simulink model "STEVE_Simulation"  (R2024b)
settings: Solver=ode8  StartTime=0.0  StopTime=Sim.Time  FixedStep=Sim.Timestep  RelTol=1e-3  EnableMultiTasking=on
values from neighbouring files (symbols this model uses):
  AeroData = CombinedAeroData    [initialize_sim_parameters.m]
  m = 1277.9    [LQR_Controller_Design.m]    (also in controlability_analysis.m = params.mass(i); lqr_gain_scedule.m = interp_data.mass(i); matlab.mat = 974)
  q = 0.5 * rho * V^2    (= 29036.16)    [LQR_Controller_Design.m]    (also in matlab.mat = 2919.616)
  Ref_Area = RocketAeroPhysical.Reference_Area    [initialize_sim_parameters.m]
undefined symbols (not defined in the file or in its folder): Actuators, Earth, F, Initial, Light, MIL, PrelookupData, rocket_length, RocketAeroPhysical, s, ThrustLookupData, timeStep, WGS84
libraries: simulink x6, simulink_extras x4, aerolibwind2 x4, aerolibtransform2 x3, aerolibasang x3, aerolibconvert2 x2, aerolibnav x2, aerolibactuator x2, aerolibatmos2 x1, dspsrcs4 x1, mspfiltlib x1, sharedtransform x1
(part 1 of 2)
settings Model: SimulationMode=accelerator  ExtModeTrigDuration=2  Creator=jonno  LastModifiedBy=jonno
settings SolverCC: AutoInsertRateTranBlk=on
settings HardwareCC: ProdBitPerLong=64  ProdHWDeviceType=Apple->ARM64
settings RTWCC: BuildConfiguration=Faster Runs
settings GRTTargetCC: RTWCAPISignals=on  RTWCAPIParams=on

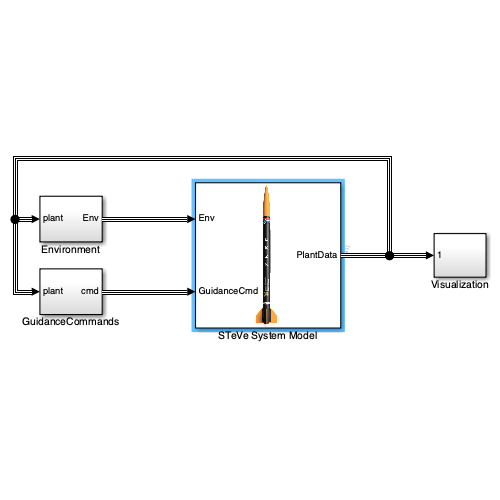
[thumbnail: Simulink's stored preview of the top-level diagram]
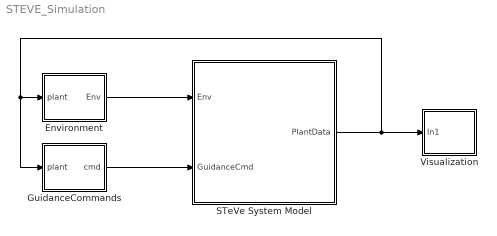
== system STEVE_Simulation ==
  Environment : Subsystem
  GuidanceCommands : Subsystem
  STeVe System Model : Subsystem
      mask Display: image('/Users/jonno/MATLAB-Drive/Rocket-Model-Simulation/STEVE_Simulator/docs/images/steve.png', [65 - (50 * (187 / 1041)), 0, 140 * (187 / 1041), 140])
  Visualization : Subsystem
  wires:
  GuidanceCommands/1(cmd) -> STeVe System Model/2(GuidanceCmd)
  Environment/1(Env) -> STeVe System Model/1(Env)
  STeVe System Model/1(PlantData) -> GuidanceCommands/1(plant), Environment/1(plant), Visualization/1(In1)

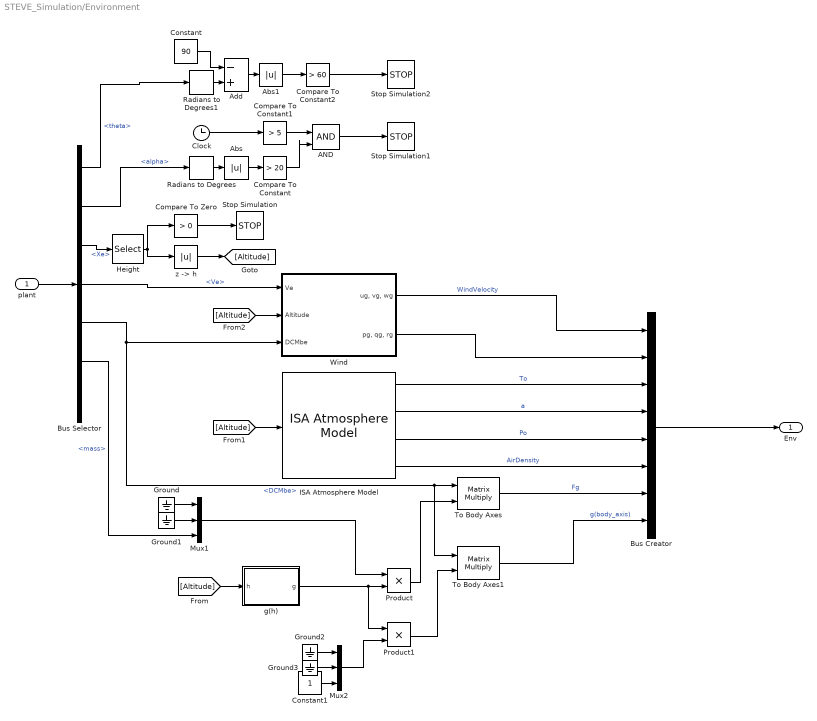
== system STEVE_Simulation/Environment ==
  plant : Inport
  AND : Logic  IconShape=distinctive  AllPortsSameDT=off  OutDataTypeStr=boolean
  Abs : Abs  SaturateOnIntegerOverflow=off
  Abs1 : Abs  SaturateOnIntegerOverflow=off
  Add : Sum  Inputs=-+
  Bus Creator : BusCreator  Inputs=8
  Bus Selector : BusSelector  OutputSignals=body angles.theta,alpha,Xe,Ve,DCMbe,mass,lat
  Clock : Clock
  Compare To Constant : simulink/Logic and Bit Operations/Compare To Constant  relop=>  const=20  OutDataTypeStr=boolean
  Compare To Constant1 : simulink/Logic and Bit Operations/Compare To Constant  relop=>  const=5  OutDataTypeStr=boolean
  Compare To Constant2 : simulink/Logic and Bit Operations/Compare To Constant  relop=>  const=60  OutDataTypeStr=boolean
  Compare To Zero : simulink/Logic and Bit Operations/Compare To Zero  relop=>  OutDataTypeStr=boolean
  Constant : Constant  Value=90
  Constant1 : Constant
  Ground{,1..3} (4 alike) : Ground
  Height : Selector  IndexMode=Zero-based  InputPortWidth=3  IndexOptions=Index vector (dialog)  Indices=2  OutputSizes=1
  ISA Atmosphere Model : aerolibatmos2/ISA Atmosphere Model  useExtended=on  action=None  custom=off  viscosityOut=off  g=9.80665  gamma=1.4  R=287.0531  L=0.0065  h_trop=11000  h_strat=20000  rho0=1.225  P0=101325  T0=288.15  h0=0  S=110.4  Tref=273.15  muref=1.716e-5
  Mux1 : Mux  Inputs=3
  Mux2 : Mux  Inputs=3
  Product : Product
  Product1 : Product
  Radians to Degrees : simulink_extras/Transformations/Radians to Degrees
  Radians to Degrees1 : simulink_extras/Transformations/Radians to Degrees
  Stop Simulation : Stop
  Stop Simulation1 : Stop
  Stop Simulation2 : Stop
  To Body Axes : Product  Multiplication=Matrix(*)
  To Body Axes1 : Product  Multiplication=Matrix(*)
  Wind : Subsystem
  g(h) : MATLAB Function  TreatAsAtomicUnit=on
  "z -> h" : Abs  SaturateOnIntegerOverflow=off
  Env : Outport
  wires:
  plant/1 -> Bus Selector/1
  Bus Creator/1 -> Env/1
  Bus Selector/3 -> Height/1  "<Xe>"
  Height/1 -> Compare To Zero/1, "z -> h"/1
  "z -> h"/1 -> [Altitude]
  Bus Selector/6 -> Mux1/3  "<mass>"
  Ground/1 -> Mux1/1
  Ground1/1 -> Mux1/2
  Bus Selector/5 -> Wind/3(DCMbe), To Body Axes1/1, To Body Axes/1  "<DCMbe>"
  [Altitude] -> ISA Atmosphere Model/1
  To Body Axes/1 -> Bus Creator/7  "Fg"
  ISA Atmosphere Model/4 -> Bus Creator/6  "AirDensity"
  ISA Atmosphere Model/3 -> Bus Creator/5  "Po"
  ISA Atmosphere Model/2 -> Bus Creator/4  "a"
  ISA Atmosphere Model/1 -> Bus Creator/3  "To"
  Bus Selector/4 -> Wind/1(Ve)  "<Ve>"
  [Altitude] -> Wind/2(Altitude)
  Wind/2("pg, qg, rg") -> Bus Creator/2
  Mux1/1 -> Product/1
  Product/1 -> To Body Axes/2
  [Altitude] -> g(h)/1(h)
  g(h)/1(g) -> Product1/1, Product/2
  Wind/1("ug, vg, wg") -> Bus Creator/1  "WindVelocity"
  Bus Selector/2 -> Radians to Degrees/1  "<alpha>"
  Compare To Zero/1 -> Stop Simulation/1
  AND/1 -> Stop Simulation1/1
  Compare To Constant/1 -> AND/2
  Compare To Constant1/1 -> AND/1
  Clock/1 -> Compare To Constant1/1
  Radians to Degrees/1 -> Abs/1
  Abs/1 -> Compare To Constant/1
  Bus Selector/1 -> Radians to Degrees1/1  "<theta>"
  Radians to Degrees1/1 -> Add/2
  Constant/1 -> Add/1
  Add/1 -> Abs1/1
  Abs1/1 -> Compare To Constant2/1
  Compare To Constant2/1 -> Stop Simulation2/1
  Ground2/1 -> Mux2/1
  Ground3/1 -> Mux2/2
  Constant1/1 -> Mux2/3
  Mux2/1 -> Product1/2
  Product1/1 -> To Body Axes1/2
  To Body Axes1/1 -> Bus Creator/8  "g(body_axis)"

== system STEVE_Simulation/GuidanceCommands ==
  plant : Inport
  Add : Sum  Inputs=+++
  Bus Creator : BusCreator  Inputs=2
  Constant : Constant  Value=85
  Degrees to Radians : simulink_extras/Transformations/Degrees to Radians
  Rate Limiter : RateLimiter  RisingSlewLimit=Initial.Conditions.pitchRate  FallingSlewLimit=-Initial.Conditions.pitchRate  SampleTimeMode=inherited
  Rate Limiter1 : RateLimiter  RisingSlewLimit=20  FallingSlewLimit=-20  SampleTimeMode=inherited
  Rate Limiter2 : RateLimiter  RisingSlewLimit=0.1  FallingSlewLimit=-0.1  SampleTimeMode=inherited
  Rate Limiter3 : RateLimiter  SampleTimeMode=inherited
  Scope : Scope
  ThetaCmd : Step  Time=8  After=90 - Initial.Conditions.tiltAngle*180/pi  SampleTime=0
  ThetaCmd1 : Step  Time=0.5  Before=90  After=Initial.Conditions.tiltAngle*180/pi  SampleTime=0
  ThetaCmd2 : Step  Time=65  After=0  SampleTime=0
  ThrottleCmd %1 : Step  Time=Actuators.Engine.BurnTime  Before=1  After=0.05  SampleTime=0  VectorParams1D=off
  To Workspace : ToWorkspace  VariableName=thetaCmd  SaveFormat=Timeseries  SampleTime=-1
  cmd : Outport
  wires:
  Bus Creator/1 -> cmd/1
  ThetaCmd/1 -> Rate Limiter/1  "ThetaCmd"
  Degrees to Radians/1 -> Scope/1, To Workspace/1, Bus Creator/2  "ThetaCmd"
  ThrottleCmd %1/1 -> Rate Limiter2/1  "ThrottleCmd"
  Rate Limiter/1 -> Add/1
  ThetaCmd1/1 -> Rate Limiter1/1  "ThetaCmd"
  Rate Limiter1/1 -> Add/2
  Rate Limiter2/1 -> Bus Creator/1  "ThrottleCmd"
  ThetaCmd2/1 -> Rate Limiter3/1  "ThetaCmd"
  Rate Limiter3/1 -> Add/3
  Constant/1 -> Degrees to Radians/1

== system STEVE_Simulation/STeVe System Model ==
  Env : Inport
  GuidanceCmd : Inport  Port=2
  Avionics : Subsystem
  Env1 : InportShadow
  Flight Sensors : Subsystem
  Vehicle Dynamics : Subsystem
  PlantData : Outport
  wires:
  Env/1 -> Vehicle Dynamics/1(Env)
  Vehicle Dynamics/1(PlantData) -> Flight Sensors/2(Plant), Avionics/3(PlantData), PlantData/1  "Plant"
  Avionics/1(ActCmd) -> Vehicle Dynamics/2(ActCmd)
  GuidanceCmd/1 -> Avionics/1(GuidanceCommandBus)
  Env1/1 -> Flight Sensors/1(Env)
  Flight Sensors/1(Sensors) -> Avionics/2(Sensors)

== system STEVE_Simulation/Visualization ==
  In1 : Inport
  Bus Selector : BusSelector  OutputSignals=Xe
  Bus Selector1 : BusSelector  OutputSignals=Ve,Xe,Vb,body angles.phi,body angles.theta,body angles.psi,alpha,lat,long,alt,w
  Demux : Demux  Outputs=3
  In2 : InportShadow
  Multiply : Gain  Gain=-1
  To Workspace : ToWorkspace  VariableName=Ve  SaveFormat=Timeseries  SampleTime=-1
  To Workspace1 : ToWorkspace  VariableName=Xe  SaveFormat=Timeseries  SampleTime=-1
  To Workspace10 : ToWorkspace  VariableName=w  SaveFormat=Timeseries  SampleTime=-1
  To Workspace2 : ToWorkspace  VariableName=Vb  SaveFormat=Timeseries  SampleTime=-1
  To Workspace3 : ToWorkspace  VariableName=phi  SaveFormat=Timeseries  SampleTime=-1
  To Workspace4 : ToWorkspace  VariableName=theta  SaveFormat=Timeseries  SampleTime=-1
  To Workspace5 : ToWorkspace  VariableName=psi  SaveFormat=Timeseries  SampleTime=-1
  To Workspace6 : ToWorkspace  VariableName=alpha  SaveFormat=Timeseries  SampleTime=-1
  To Workspace7 : ToWorkspace  VariableName=lat  SaveFormat=Timeseries  SampleTime=-1
  To Workspace8 : ToWorkspace  VariableName=long  SaveFormat=Timeseries  SampleTime=-1
  To Workspace9 : ToWorkspace  VariableName=alt  SaveFormat=Timeseries  SampleTime=-1
  XY Graph : Record  FileSettingsInternal="{\"entries\":[{\"content\":{\"excelSettings\":{\"content\":{},\"type\":\"Streamout.ExcelSettings\"}},\"type\":\"Streamout.FileSettingStorage\",\"uuid\":\"\"}],\"packageUris\":[\"http:\\/\\/schema.mathworks.com\\/mf0\\/streamout_blocks\\/R2020a\"],\"version\":\"1.0\"}"  Layout=[1 1]  SignalsInternal="{\"entries\":[{\"content\":{\"signals\":[{\"content\":{\"blockPath\":[],\"dimensions\":[1],\"domain\":\"\",\"lineColor\":\"#a2142f\",\"plots\":[ 1 ],\"port\":1,\"signalID\":1,\"signalName\":\"Demux:1\"},\"type\":\"RecordBlkView.Signal\",\"uuid\":\"\"},{\"content\":{\"blockPath\":[],\"dimensions\":[1],\"domain\":\"\",\"lineColor\":\"#139fff\",\"plots\":[ 1 ],\"port\":2,\"signalID\":2,\"signalName\":\"Multiply\"},\"type\":\"RecordBlkView.Signal\",\"uuid\":\"\"}]},\"type\":\"RecordBlkView.InputSignals\",\"uuid\":\"\"}],\"packageUris\":[\"http:\\/\\/schema.mathworks.com\\/mf0\\/streamout_blocks\\/R2020a\"],\"version\":\"1.0\"}"  VisualizationBindings="{\"xyplotplugin\":{\"info\":[{\"series\":[{\"bindingParametersList\":[{\"parameter\":\"X-Axis\",\"signalID\":1,\"signalName\":\"Demux:1\"},{\"parameter\":\"Y-Axis\",\"signalID\":2,\"signalName\":\"Multiply\"}],\"seriesID\":0}],\"subplotID\":1}]}}"  CompatibilityTag=XY
  wires:
  In1/1 -> Bus Selector/1
  Bus Selector/1 -> Demux/1  "<Xe>"
  Multiply/1 -> XY Graph/2
  Demux/3 -> Multiply/1
  Demux/1 -> XY Graph/1
  In2/1 -> Bus Selector1/1
  Bus Selector1/1 -> To Workspace/1  "<Ve>"
  Bus Selector1/2 -> To Workspace1/1  "<Xe>"
  Bus Selector1/3 -> To Workspace2/1  "<Vb>"
  Bus Selector1/4 -> To Workspace3/1  "<phi>"
  Bus Selector1/5 -> To Workspace4/1  "<theta>"
  Bus Selector1/6 -> To Workspace5/1  "<psi>"
  Bus Selector1/7 -> To Workspace6/1  "<alpha>"
  Bus Selector1/8 -> To Workspace7/1  "<lat>"
  Bus Selector1/9 -> To Workspace8/1  "<long>"
  Bus Selector1/10 -> To Workspace9/1  "<alt>"
  Bus Selector1/11 -> To Workspace10/1  "<w>"

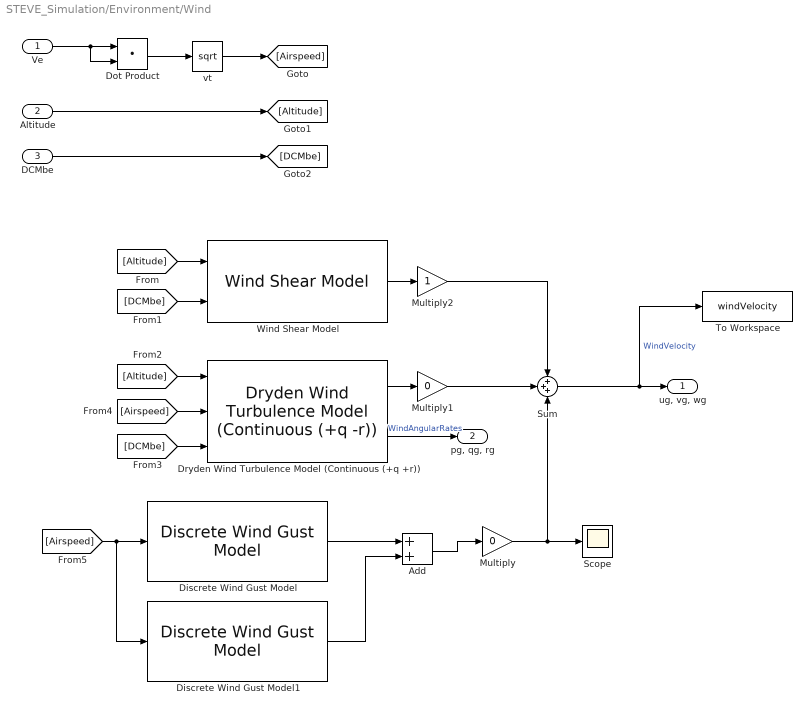
== system STEVE_Simulation/Environment/Wind ==
  Ve : Inport
  Altitude : Inport  Port=2
  DCMbe : Inport  Port=3
  Add : Sum
  Discrete Wind Gust Model : aerolibwind2/Discrete Wind Gust Model  units=Metric (MKS)  Gx=on  Gy=on  Gz=on  t_0=1  d_m=[2 2 5]  v_m=[0 0 -30]
  Discrete Wind Gust Model1 : aerolibwind2/Discrete Wind Gust Model  units=Metric (MKS)  Gx=on  Gy=on  Gz=on  t_0=2  d_m=[2 2 5]  v_m=[0 0 30]
  Dot Product : DotProduct  OutDataTypeStr=Inherit: Inherit via internal rule
  Dryden Wind Turbulence Model (Continuous (+q +r)) : aerolibwind2/Dryden Wind Turbulence Model  (Continuous (+q -r))  units=Metric (MKS)  spec=MIL-F-8785C  model=Continuous Dryden (+q +r)  W20=15  Wdeg=0  TurbProb=10^-2 - Light  L_high=533.4  Wingspan=10  ts=0.1  Seed=[23341 23342 23343 23344]  T_on=off
      settings: LibrarySourceBlock=|
      | aerolibwind2/Dryden Wind Turbulence Model
      | (Continuous (+q +r))
  Multiply : Gain  Gain=0
  Multiply1 : Gain  Gain=0
  Multiply2 : Gain
  Scope : Scope
  Sum : Sum  Inputs=+++
  To Workspace : ToWorkspace  VariableName=windVelocity  SaveFormat=Timeseries  SampleTime=-1
  Wind Shear Model : aerolibwind2/Wind Shear Model  units=Metric (MKS)  phase=Category C - Terminal Flight Phase  W_20=Wind.shear  Wdeg=90
  vt : Sqrt
  "ug, vg, wg" : Outport
  "pg, qg, rg" : Outport  Port=2
  wires:
  Ve/1 -> Dot Product/2, Dot Product/1
  Dot Product/1 -> vt/1
  vt/1 -> [Airspeed]
  DCMbe/1 -> [DCMbe]
  [Altitude] -> Wind Shear Model/1
  [DCMbe] -> Wind Shear Model/2
  [Altitude] -> Dryden Wind Turbulence Model (Continuous (+q +r))/1
  [DCMbe] -> Dryden Wind Turbulence Model (Continuous (+q +r))/3
  [Airspeed] -> Dryden Wind Turbulence Model (Continuous (+q +r))/2
  [Airspeed] -> Discrete Wind Gust Model1/1, Discrete Wind Gust Model/1
  Discrete Wind Gust Model/1 -> Add/1
  Sum/1 -> To Workspace/1, "ug, vg, wg"/1  "WindVelocity"
  Dryden Wind Turbulence Model (Continuous (+q +r))/2 -> "pg, qg, rg"/1  "WindAngularRates"
  Altitude/1 -> [Altitude]
  Multiply/1 -> Sum/3, Scope/1
  Wind Shear Model/1 -> Multiply2/1
  Dryden Wind Turbulence Model (Continuous (+q +r))/1 -> Multiply1/1
  Multiply1/1 -> Sum/2
  Multiply2/1 -> Sum/1
  Discrete Wind Gust Model1/1 -> Add/2
  Add/1 -> Multiply/1

== system STEVE_Simulation/STeVe System Model/Avionics ==
  GuidanceCommandBus : Inport
  Sensors : Inport  Port=2
  PlantData : Inport  Port=3
  Bus Selector : BusSelector  OutputSignals=Ve,body angles.theta,w
  Compare To Zero : simulink/Logic and Bit Operations/Compare To Zero  relop=>  OutDataTypeStr=boolean
  ControlSystem : Subsystem
  Delay : Delay  DelayLength=10
  Selector : Selector  InputPortWidth=3  IndexOptions=Index vector (dialog)  Indices=3  OutputSizes=1
  Stop Simulation : Stop
  ActCmd : Outport
  wires:
  PlantData/1 -> Bus Selector/1, ControlSystem/1(AvionicsBus)
  GuidanceCommandBus/1 -> ControlSystem/2(Guidance)
  ControlSystem/1(cmd) -> ActCmd/1
  Sensors/1 -> ?
  Bus Selector/1 -> Selector/1  "<Ve>"
  Selector/1 -> Compare To Zero/1
  Compare To Zero/1 -> Delay/1
  Delay/1 -> Stop Simulation/1

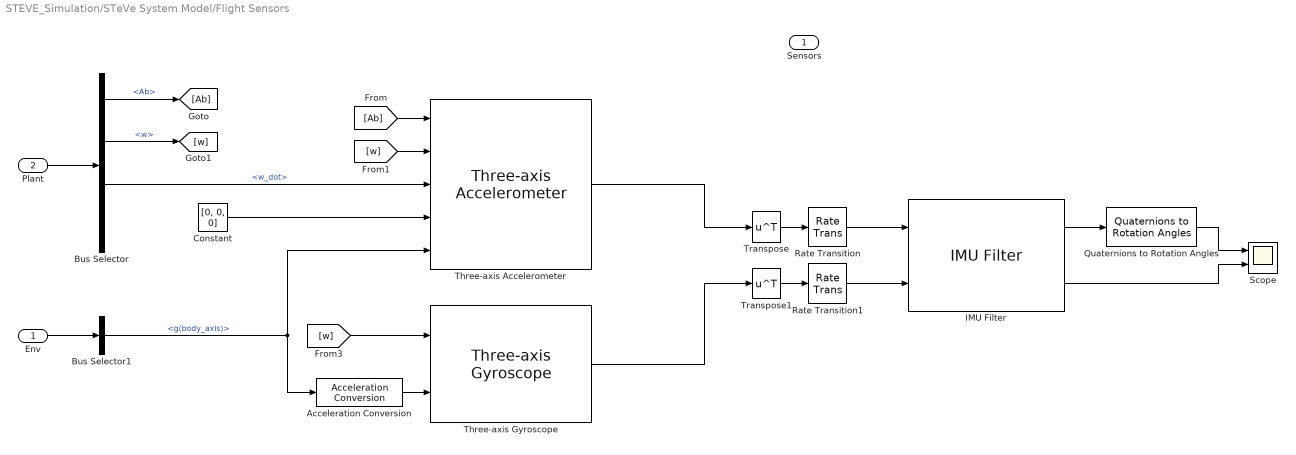
== system STEVE_Simulation/STeVe System Model/Flight Sensors ==
  Env : Inport
  Plant : Inport  Port=2
  Acceleration Conversion : aerolibconvert2/Acceleration Conversion  IU=m/s^2  OU=G's
  Bus Selector : BusSelector  OutputSignals=Ab,w,w_dot,DCMbe
  Bus Selector1 : BusSelector  OutputSignals=g(body_axis)
  Constant : Constant  Value=[0, 0, 0]
  IMU Filter : mspfiltlib/IMU Filter  DispRefFrame=NED  OrientationFormat=quaternion  DecimationFactor=1  InitialProcessNoise=imufilter.defaultProcessNoise  AccelerometerNoise=0.0001924722  GyroscopeNoise=9.1385e-5  GyroscopeDriftNoise=3.0462e-13  LinearAccelerationNoise=0.0096236100000000012  LinearAccelerationDecayFactor=0.5  SimulateUsing=Interpreted execution
  Quaternions to Rotation Angles : sharedtransform/Quaternions to Rotation Angles  rotationOrder=ZYX  aMode=aMode
  Rate Transition : RateTransition
  Rate Transition1 : RateTransition
  Scope : Scope  NumInputPorts=2
  Three-axis Accelerometer : aerolibnav/Three-axis Accelerometer  units=Metric (MKS)  acc=[0 0 0]  gtype=on  dtype_a=on  w_a=190  z_a=0.707  a_sf_cc=[1 0 0; 0 1 0; 0 0 1]  a_bias=[0 0 0]  a_Ts=0  a_rand=off  a_seeds=[23093 23094 23095]  a_pow=[0.001 0.001 0.001]  a_sat="[-inf  -inf  -inf  inf inf inf]"
  Three-axis Gyroscope : aerolibnav/Three-axis Gyroscope  dtype_g=on  w_g=190  z_g=0.707  g_sf_cc=[1 0 0; 0 1 0; 0 0 1]  g_bias=[0 0 0]  g_sen=[0 0 0]  g_Ts=0  g_rand=off  g_seeds=[23093 23094 23095]  g_pow=[0.0001 0.0001 0.0001]  g_sat="[-inf  -inf  -inf  inf inf inf]"
  Transpose : Math  Operator=transpose
  Transpose1 : Math  Operator=transpose
  Sensors : Outport
  wires:
  Plant/1 -> Bus Selector/1
  Bus Selector/1 -> [Ab]  "<Ab>"
  Bus Selector/2 -> [w]  "<w>"
  Bus Selector/3 -> Three-axis Accelerometer/3  "<w_dot>"
  Constant/1 -> Three-axis Accelerometer/4
  Env/1 -> Bus Selector1/1
  Bus Selector1/1 -> Acceleration Conversion/1, Three-axis Accelerometer/5  "<g(body_axis)>"
  [Ab] -> Three-axis Accelerometer/1
  [w] -> Three-axis Accelerometer/2
  [w] -> Three-axis Gyroscope/1
  Acceleration Conversion/1 -> Three-axis Gyroscope/2
  Three-axis Accelerometer/1 -> Transpose/1
  Three-axis Gyroscope/1 -> Transpose1/1
  Transpose/1 -> Rate Transition/1
  Transpose1/1 -> Rate Transition1/1
  Rate Transition/1 -> IMU Filter/1
  Rate Transition1/1 -> IMU Filter/2
  IMU Filter/2 -> Scope/2
  IMU Filter/1 -> Quaternions to Rotation Angles/1
  Quaternions to Rotation Angles/1 -> Scope/1

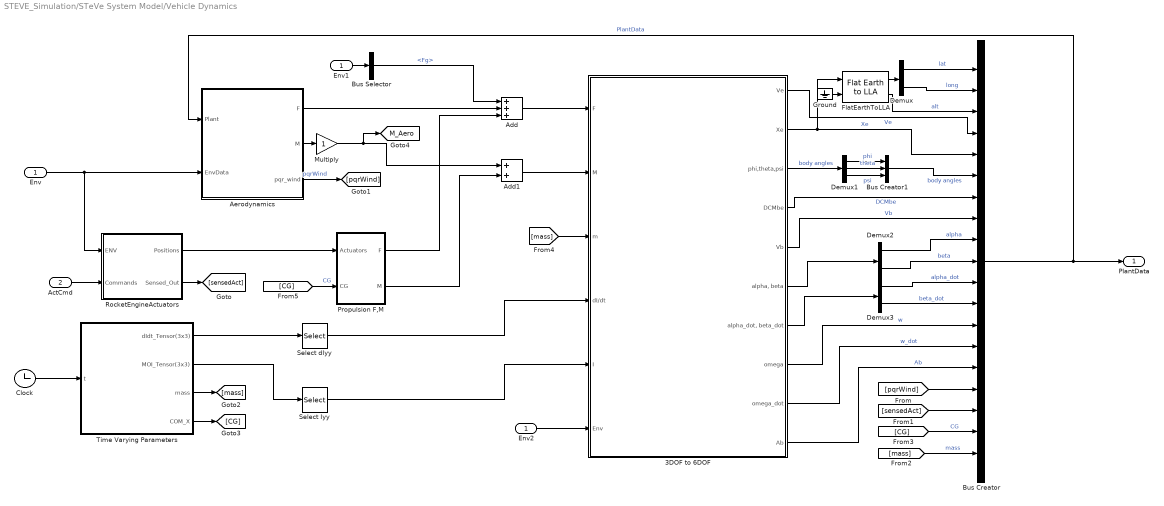
== system STEVE_Simulation/STeVe System Model/Vehicle Dynamics ==
  Env : Inport
  ActCmd : Inport  Port=2
  3DOF to 6DOF : Subsystem
  Add : Sum  Inputs=+++
  Add1 : Sum
  Aerodynamics : Subsystem
  Bus Creator : BusCreator  Inputs=19
  Bus Creator1 : BusCreator  Inputs=3
  Bus Selector : BusSelector  OutputSignals=Fg
  Clock : Clock
  Demux : Demux  Outputs=2
  Demux1 : Demux  Outputs=3
  Demux2 : Demux  Outputs=2
  Demux3 : Demux  Outputs=2
  Env1 : InportShadow
  Env2 : InportShadow
  FlatEarthToLLA : aerolibtransform2/Flat Earth to LLA  units=Metric (MKS)  ptype=Earth (WGS84)  F=1/298.257223563  R=6378137  refPosPort=off  LL0=[0 10]  psi=0
  Ground : Ground
  Multiply : Gain
  Propulsion F,M : Subsystem
  RocketEngineActuators : Subsystem
  Select Iyy : Selector  NumberOfDimensions=2  InputPortWidth=3  IndexOptions=Index vector (dialog),Index vector (dialog)  Indices=[1],[1]  OutputSizes=1,1
  Select dIyy : Selector  NumberOfDimensions=2  InputPortWidth=3  IndexOptions=Index vector (dialog),Index vector (dialog)  Indices=[1],[1]  OutputSizes=1,1
  Time Varying Parameters : Subsystem
  PlantData : Outport
  tag scope: M_Aero=global
  wires:
  ActCmd/1 -> RocketEngineActuators/2(Commands)
  RocketEngineActuators/1(Positions) -> Propulsion F,M/1(Actuators)
  Bus Creator/1 -> Aerodynamics/1(Plant), PlantData/1  "PlantData"
  3DOF to 6DOF/2(Xe) -> FlatEarthToLLA/1, Bus Creator/5  "Xe"
  Demux/1 -> Bus Creator/1  "lat"
  Demux/2 -> Bus Creator/2  "long"
  FlatEarthToLLA/1 -> Demux/1
  FlatEarthToLLA/2 -> Bus Creator/3  "alt"
  Ground/1 -> FlatEarthToLLA/2
  3DOF to 6DOF/1(Ve) -> Bus Creator/4  "Ve"
  3DOF to 6DOF/3(phi,theta,psi) -> Demux1/1  "body angles"
  Demux1/1 -> Bus Creator1/1  "phi"
  Demux1/2 -> Bus Creator1/2  "theta"
  Demux1/3 -> Bus Creator1/3  "psi"
  Bus Creator1/1 -> Bus Creator/6  "body angles"
  3DOF to 6DOF/4(DCMbe) -> Bus Creator/7  "DCMbe"
  3DOF to 6DOF/5(Vb) -> Bus Creator/8  "Vb"
  3DOF to 6DOF/6("alpha, beta") -> Demux2/1
  Demux2/1 -> Bus Creator/9  "alpha"
  Demux2/2 -> Bus Creator/10  "beta"
  Demux3/2 -> Bus Creator/12  "beta_dot"
  Demux3/1 -> Bus Creator/11  "alpha_dot"
  3DOF to 6DOF/7("alpha_dot, beta_dot") -> Demux3/1
  3DOF to 6DOF/8(omega) -> Bus Creator/13  "w"
  3DOF to 6DOF/9(omega_dot) -> Bus Creator/14  "w_dot"
  3DOF to 6DOF/10(Ab) -> Bus Creator/15  "Ab"
  [pqrWind] -> Bus Creator/16
  [sensedAct] -> Bus Creator/17
  RocketEngineActuators/2(Sensed_Out) -> [sensedAct]
  Aerodynamics/3(pqr_wind) -> [pqrWind]  "pqrWind"
  Propulsion F,M/1(F) -> Add/3
  [CG] -> Bus Creator/18  "CG"
  [mass] -> Bus Creator/19  "mass"
  Env1/1 -> Bus Selector/1
  Bus Selector/1 -> Add/1  "<Fg>"
  Env/1 -> RocketEngineActuators/1(ENV), Aerodynamics/2(EnvData)
  Propulsion F,M/2(M) -> Add1/2
  Clock/1 -> Time Varying Parameters/1(t)
  Time Varying Parameters/1(dIdt_Tensor(3x3)) -> Select dIyy/1
  Select dIyy/1 -> 3DOF to 6DOF/4(dI/dt)
  Time Varying Parameters/2(MOI_Tensor(3x3)) -> Select Iyy/1
  Select Iyy/1 -> 3DOF to 6DOF/5(I)
  Time Varying Parameters/3(mass) -> [mass]
  Time Varying Parameters/4(COM_X) -> [CG]
  [mass] -> 3DOF to 6DOF/3(m)
  Add1/1 -> 3DOF to 6DOF/2(M)
  Add/1 -> 3DOF to 6DOF/1(F)
  Aerodynamics/1(F) -> Add/2
  Env2/1 -> 3DOF to 6DOF/6(Env)
  [CG] -> Propulsion F,M/2(CG)  "CG"
  Aerodynamics/2(M) -> Multiply/1
  Multiply/1 -> Add1/1, [M_Aero]

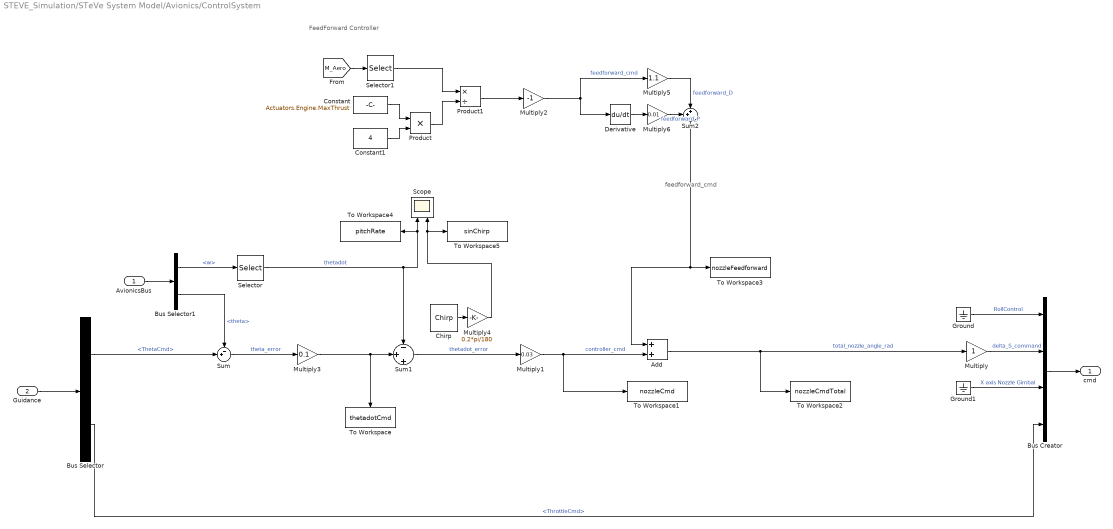
== system STEVE_Simulation/STeVe System Model/Avionics/ControlSystem ==
  note: feedforward_cmd
  note: FeedForward Controller
  AvionicsBus : Inport
  Guidance : Inport  Port=2
  Add : Sum
  Bus Creator : BusCreator  Inputs=4
  Bus Selector : BusSelector  OutputSignals=ThetaCmd,ThrottleCmd
  Bus Selector1 : BusSelector  OutputSignals=w,body angles.theta
  Chirp : dspsrcs4/Chirp  sweep=Logarithmic  mode=Unidirectional  f0=1  f1=50  t1=20  Tsweep=20  phase=0  Ts=0.0001  spf=1  datatype=double  OutputFrames=off
  Constant : Constant  Value=Actuators.Engine.MaxThrust
  Constant1 : Constant  Value=4
  Derivative : Derivative
  Ground : Ground
  Ground1 : Ground
  Multiply : Gain
  Multiply1 : Gain  Gain=0.03
  Multiply2 : Gain  Gain=-1
  Multiply3 : Gain  Gain=0.1
  Multiply4 : Gain  Gain=0.2*pi/180
  Multiply5 : Gain  Gain=1.1
  Multiply6 : Gain  Gain=0.01
  Product : Product
  Product1 : Product  Inputs=*/
  Scope : Scope  NumInputPorts=2
  Selector : Selector  InputPortWidth=3  IndexOptions=Index vector (dialog)  Indices=2  OutputSizes=1
  Selector1 : Selector  InputPortWidth=3  IndexOptions=Index vector (dialog)  Indices=[2]  OutputSizes=1
  Sum : Sum  Inputs=-+|
  Sum1 : Sum  Inputs=-|+|+
  Sum2 : Sum  Inputs=++|
  To Workspace : ToWorkspace  VariableName=thetadotCmd  SaveFormat=Timeseries  SampleTime=-1
  To Workspace1 : ToWorkspace  VariableName=nozzleCmd  SaveFormat=Timeseries  SampleTime=-1
  To Workspace2 : ToWorkspace  VariableName=nozzleCmdTotal  SaveFormat=Timeseries  SampleTime=-1
  To Workspace3 : ToWorkspace  VariableName=nozzleFeedforward  SaveFormat=Timeseries  SampleTime=-1
  To Workspace4 : ToWorkspace  VariableName=pitchRate  SaveFormat=Timeseries  SampleTime=-1
  To Workspace5 : ToWorkspace  VariableName=sinChirp  SaveFormat=Timeseries  SampleTime=-1
  cmd : Outport
  wires:
  Bus Creator/1 -> cmd/1
  Ground/1 -> Bus Creator/1  "RollControl"
  Ground1/1 -> Bus Creator/3  "X axis Nozzle Gimbal"
  Guidance/1 -> Bus Selector/1
  Bus Selector/2 -> Bus Creator/4  "<ThrottleCmd>"
  Bus Selector/1 -> Sum/2  "<ThetaCmd>"
  AvionicsBus/1 -> Bus Selector1/1
  Bus Selector1/1 -> Selector/1  "<w>"
  Multiply/1 -> Bus Creator/2  "delta_S_command"
  Sum1/1 -> Multiply1/1  "thetadot_error"
  Selector/1 -> To Workspace4/1, Scope/1, Sum1/1  "thetadot"
  Bus Selector1/2 -> Sum/1  "<theta>"
  Sum/1 -> Multiply3/1  "theta_error"
  Constant1/1 -> Product/2
  Constant/1 -> Product/1
  Product/1 -> Product1/2
  [M_Aero] -> Selector1/1
  Selector1/1 -> Product1/1
  Multiply4/1 -> To Workspace5/1, Scope/2
  Add/1 -> Multiply/1, To Workspace2/1  "total_nozzle_angle_rad"
  Product1/1 -> Multiply2/1
  Multiply3/1 -> To Workspace/1, Sum1/2
  Chirp/1 -> Multiply4/1
  Multiply1/1 -> To Workspace1/1, Add/2  "controller_cmd"
  Multiply2/1 -> Derivative/1, Multiply5/1  "feedforward_cmd"
  Derivative/1 -> Multiply6/1
  Multiply5/1 -> Sum2/2  "feedforward_D"
  Multiply6/1 -> Sum2/1  "feedforward_P"
  Sum2/1 -> Add/1, To Workspace3/1

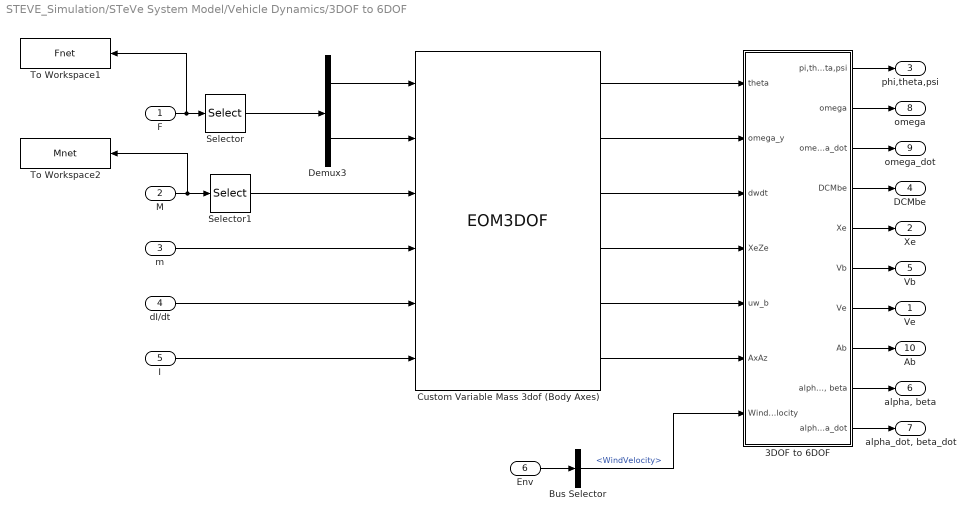
== system STEVE_Simulation/STeVe System Model/Vehicle Dynamics/3DOF to 6DOF ==
  F : Inport
  M : Inport  Port=2
  m : Inport  Port=3
  dI/dt : Inport  Port=4
  I : Inport  Port=5
  Env : Inport  Port=6
  3DOF to 6DOF : Subsystem
  Bus Selector : BusSelector  OutputSignals=WindVelocity
  Custom Variable Mass 3dof (Body Axes) : EOM3DOF  mtype=Custom Variable  v_ini=Initial.Conditions.V0  theta_ini=Initial.Conditions.theta0  pos_ini=[0 Initial.Conditions.h0]  g=0
  Demux3 : Demux  Outputs=2
  Selector : Selector  InputPortWidth=3  IndexOptions=Index vector (dialog)  Indices=[1 3]  OutputSizes=1
  Selector1 : Selector  InputPortWidth=3  IndexOptions=Index vector (dialog)  Indices=[2]  OutputSizes=1
  To Workspace1 : ToWorkspace  VariableName=Fnet  SaveFormat=Timeseries  SampleTime=-1
  To Workspace2 : ToWorkspace  VariableName=Mnet  SaveFormat=Timeseries  SampleTime=-1
  Ve : Outport
  Xe : Outport  Port=2
  phi,theta,psi : Outport  Port=3
  DCMbe : Outport  Port=4
  Vb : Outport  Port=5
  "alpha, beta" : Outport  Port=6
  "alpha_dot, beta_dot" : Outport  Port=7
  omega : Outport  Port=8
  omega_dot : Outport  Port=9
  Ab : Outport  Port=10
  wires:
  F/1 -> To Workspace1/1, Selector/1
  Demux3/2 -> Custom Variable Mass 3dof (Body Axes)/2
  Demux3/1 -> Custom Variable Mass 3dof (Body Axes)/1
  Selector/1 -> Demux3/1
  M/1 -> To Workspace2/1, Selector1/1
  Selector1/1 -> Custom Variable Mass 3dof (Body Axes)/3
  Custom Variable Mass 3dof (Body Axes)/1 -> 3DOF to 6DOF/1(theta)
  Custom Variable Mass 3dof (Body Axes)/4 -> 3DOF to 6DOF/4(XeZe)
  Custom Variable Mass 3dof (Body Axes)/6 -> 3DOF to 6DOF/6(AxAz)
  3DOF to 6DOF/1(pi,theta,psi) -> phi,theta,psi/1
  3DOF to 6DOF/2(omega) -> omega/1
  3DOF to 6DOF/3(omega_dot) -> omega_dot/1
  3DOF to 6DOF/4(DCMbe) -> DCMbe/1
  3DOF to 6DOF/5(Xe) -> Xe/1
  3DOF to 6DOF/6(Vb) -> Vb/1
  3DOF to 6DOF/7(Ve) -> Ve/1
  3DOF to 6DOF/8(Ab) -> Ab/1
  3DOF to 6DOF/9("alpha, beta") -> "alpha, beta"/1
  3DOF to 6DOF/10("alpha_dot, beta_dot") -> "alpha_dot, beta_dot"/1
  I/1 -> Custom Variable Mass 3dof (Body Axes)/6
  dI/dt/1 -> Custom Variable Mass 3dof (Body Axes)/5
  m/1 -> Custom Variable Mass 3dof (Body Axes)/4
  Custom Variable Mass 3dof (Body Axes)/2 -> 3DOF to 6DOF/2(omega_y)
  Custom Variable Mass 3dof (Body Axes)/3 -> 3DOF to 6DOF/3(dwdt)
  Custom Variable Mass 3dof (Body Axes)/5 -> 3DOF to 6DOF/5(uw_b)
  Env/1 -> Bus Selector/1
  Bus Selector/1 -> 3DOF to 6DOF/7(WindVelocity)  "<WindVelocity>"

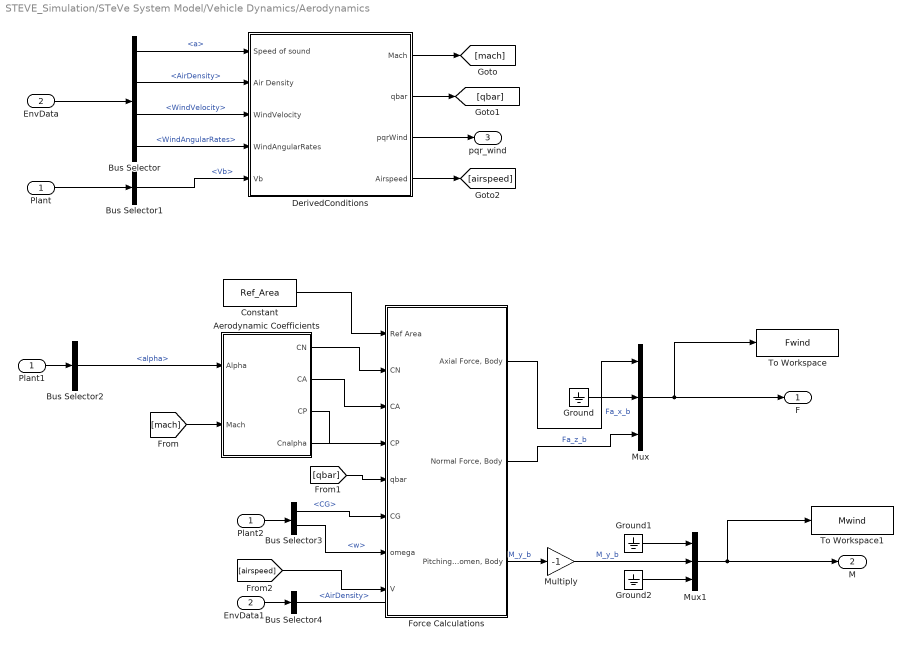
== system STEVE_Simulation/STeVe System Model/Vehicle Dynamics/Aerodynamics ==
  Plant : Inport
  EnvData : Inport  Port=2
  Aerodynamic Coefficients : Subsystem
  Bus Selector : BusSelector  OutputSignals=a,AirDensity,WindVelocity,WindAngularRates
  Bus Selector1 : BusSelector  OutputSignals=Vb
  Bus Selector2 : BusSelector  OutputSignals=alpha
  Bus Selector3 : BusSelector  OutputSignals=CG,w
  Bus Selector4 : BusSelector  OutputSignals=AirDensity
  Constant : Constant  Value=Ref_Area  VectorParams1D=off
  DerivedConditions : Subsystem
  EnvData1 : InportShadow  Port=2
  Force Calculations : Subsystem
  Ground : Ground
  Ground1 : Ground
  Ground2 : Ground
  Multiply : Gain  Gain=-1
  Mux : Mux  Inputs=3
  Mux1 : Mux  Inputs=3
  Plant1 : InportShadow
  Plant2 : InportShadow
  To Workspace : ToWorkspace  VariableName=Fwind  SaveFormat=Timeseries  SampleTime=-1
  To Workspace1 : ToWorkspace  VariableName=Mwind  SaveFormat=Timeseries  SampleTime=-1
  F : Outport
  M : Outport  Port=2
  pqr_wind : Outport  Port=3
  wires:
  Plant/1 -> Bus Selector1/1
  EnvData/1 -> Bus Selector/1
  Ground2/1 -> Mux1/3
  Ground/1 -> Mux/2
  Force Calculations/2("Normal Force, Body") -> Mux/3  "Fa_z_b"
  Multiply/1 -> Mux1/2  "M_y_b"
  Ground1/1 -> Mux1/1
  Force Calculations/1("Axial Force, Body") -> Mux/1  "Fa_x_b"
  Bus Selector1/1 -> DerivedConditions/5(Vb)  "<Vb>"
  Bus Selector/4 -> DerivedConditions/4(WindAngularRates)  "<WindAngularRates>"
  Bus Selector/3 -> DerivedConditions/3(WindVelocity)  "<WindVelocity>"
  Bus Selector/2 -> DerivedConditions/2(Air Density)  "<AirDensity>"
  Bus Selector/1 -> DerivedConditions/1(Speed of sound)  "<a>"
  DerivedConditions/1(Mach) -> [mach]
  DerivedConditions/2(qbar) -> [qbar]
  DerivedConditions/3(pqrWind) -> pqr_wind/1
  Plant1/1 -> Bus Selector2/1
  Bus Selector2/1 -> Aerodynamic Coefficients/1(Alpha)  "<alpha>"
  [mach] -> Aerodynamic Coefficients/2(Mach)
  Constant/1 -> Force Calculations/1(Ref Area)
  Aerodynamic Coefficients/1(CN) -> Force Calculations/2(CN)
  Aerodynamic Coefficients/2(CA) -> Force Calculations/3(CA)
  Aerodynamic Coefficients/3(CP) -> Force Calculations/4(CP)
  Aerodynamic Coefficients/4(Cnalpha) -> ?
  [qbar] -> Force Calculations/5(qbar)
  Plant2/1 -> Bus Selector3/1
  Bus Selector3/1 -> Force Calculations/6(CG)  "<CG>"
  Force Calculations/3("Pitching Momen, Body") -> Multiply/1  "M_y_b"
  Bus Selector3/2 -> Force Calculations/7(omega)  "<w>"
  EnvData1/1 -> Bus Selector4/1
  Bus Selector4/1 -> ?  "<AirDensity>"
  DerivedConditions/4(Airspeed) -> [airspeed]
  [airspeed] -> Force Calculations/8(V)
  Mux/1 -> To Workspace/1, F/1
  Mux1/1 -> To Workspace1/1, M/1

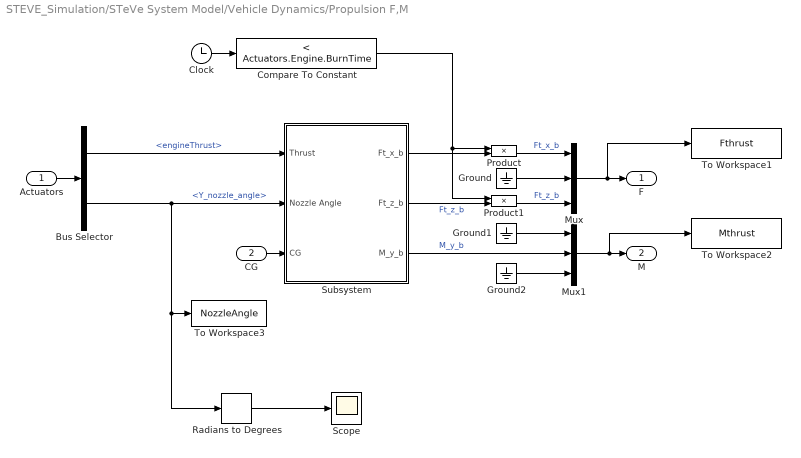
== system STEVE_Simulation/STeVe System Model/Vehicle Dynamics/Propulsion F,M ==
  Actuators : Inport
  CG : Inport  Port=2
  Bus Selector : BusSelector  OutputSignals=engineThrust,Y_nozzle_angle
  Clock : Clock
  Compare To Constant : simulink/Logic and Bit Operations/Compare To Constant  relop=<  const=Actuators.Engine.BurnTime  OutDataTypeStr=boolean
  Ground : Ground
  Ground1 : Ground
  Ground2 : Ground
  Mux : Mux  Inputs=3
  Mux1 : Mux  Inputs=3
  Product : Product  OutDataTypeStr=double
  Product1 : Product  OutDataTypeStr=double
  Radians to Degrees : simulink_extras/Transformations/Radians to Degrees
  Scope : Scope
  Subsystem : Subsystem
  To Workspace1 : ToWorkspace  VariableName=Fthrust  SaveFormat=Timeseries  SampleTime=-1
  To Workspace2 : ToWorkspace  VariableName=Mthrust  SaveFormat=Timeseries  SampleTime=-1
  To Workspace3 : ToWorkspace  VariableName=NozzleAngle  SaveFormat=Timeseries  SampleTime=-1
  F : Outport
  M : Outport  Port=2
  wires:
  Actuators/1 -> Bus Selector/1
  Bus Selector/2 -> Subsystem/2(Nozzle Angle), Radians to Degrees/1, To Workspace3/1  "<Y_nozzle_angle>"
  Bus Selector/1 -> Subsystem/1(Thrust)  "<engineThrust>"
  Subsystem/3(M_y_b) -> Mux1/2  "M_y_b"
  Subsystem/1(Ft_x_b) -> Product/2
  Product1/1 -> Mux/3  "Ft_z_b"
  Mux/1 -> To Workspace1/1, F/1
  Ground/1 -> Mux/2
  Mux1/1 -> To Workspace2/1, M/1
  Ground1/1 -> Mux1/1
  Ground2/1 -> Mux1/3
  CG/1 -> Subsystem/3(CG)
  Radians to Degrees/1 -> Scope/1
  Clock/1 -> Compare To Constant/1
  Compare To Constant/1 -> Product1/1, Product/1
  Product/1 -> Mux/1  "Ft_x_b"
  Subsystem/2(Ft_z_b) -> Product1/2  "Ft_z_b"

== system STEVE_Simulation/STeVe System Model/Vehicle Dynamics/RocketEngineActuators ==
  note: ASRI NOZZLE GIMBAL SYSTEM
  ENV : Inport
  Commands : Inport  Port=2
  1-D Lookup Table : Lookup_n-D  NumberOfTableDimensions=1  BreakpointsForDimension1=ThrustLookupData.Breakpoints.Pressure  Table=ThrustLookupData.Tables.Thrust  InternalRulePriority=Speed  RndMeth=Simplest
  Bus Creator : BusCreator  Inputs=2
  Bus Selector : BusSelector  OutputSignals=delta_S_command,ThrottleCmd
  Bus Selector1 : BusSelector  OutputSignals=Po
  Display : Display
  MATLAB Function : MATLAB Function  Commented=on  TreatAsAtomicUnit=on
  MATLAB Function1 : MATLAB Function  Commented=on  TreatAsAtomicUnit=on
  Multiply : Gain
  Nonlinear Second-Order Actuator : aerolibactuator/Nonlinear Second-Order Actuator  Commented=on  wn_fin=27*3  z_fin=0.7  fin_max=0.035  fin_min=-0.035  fin_maxrate=0.133  fin_act_0=0  fin_act_vel=0
  Product : Product
  Scope1 : Scope  NumInputPorts=2
  Servo : aerolibactuator/Nonlinear Second-Order Actuator  wn_fin=95  z_fin=0.7  fin_max=10*pi/180  fin_min=-10*pi/180  fin_maxrate=(500*pi/180)  fin_act_0=0  fin_act_vel=0
  To Workspace2 : ToWorkspace  VariableName=nozzleActuatorOutput  SaveFormat=Timeseries  SampleTime=-1
  Positions : Outport
  Sensed_Out : Outport  Port=2
  wires:
  Commands/1 -> Bus Selector/1
  Bus Creator/1 -> Sensed_Out/1, Positions/1  "Actuators"
  Bus Selector/2 -> Product/1  "<ThrottleCmd>"
  Servo/1 -> Scope1/2, To Workspace2/1, Bus Creator/1  "Y_nozzle_angle"
  ENV/1 -> Bus Selector1/1
  Bus Selector1/1 -> 1-D Lookup Table/1  "<Po>"
  1-D Lookup Table/1 -> Product/2
  Product/1 -> Display/1, Bus Creator/2  "engineThrust"
  Bus Selector/1 -> Servo/1, Multiply/1  "<delta_S_command>"
  Multiply/1 -> Scope1/1  "nozzle_angle_command"
  MATLAB Function1/1(delta_S_command) -> Nonlinear Second-Order Actuator/1
  Nonlinear Second-Order Actuator/1 -> MATLAB Function/1(delta_S)

== system STEVE_Simulation/STeVe System Model/Vehicle Dynamics/Time Varying Parameters ==
  t : Inport
  Direct Lookup Table (n-D) : LookupNDDirect  NumberOfTableDimensions=3  InputsSelectThisObjectFromTable=2-D Matrix  Table=PrelookupData.Tables.InertialTensor  DiagnosticForOutOfRangeInput=None  TableDataTypeStr=double
  Direct Lookup Table (n-D)1 : LookupNDDirect  NumberOfTableDimensions=3  InputsSelectThisObjectFromTable=2-D Matrix  Table=PrelookupData.Tables.dInertialTensor  DiagnosticForOutOfRangeInput=None  TableDataTypeStr=double
  Display : Display
  Lookup_COM_X : Interpolation_n-D  NumberOfTableDimensions=1  Table=PrelookupData.Tables.COM_X  ExtrapMethod=Clip  DiagnosticForOutOfRangeInput=Warning  RequireIndexFractionAsBus=on  InternalRulePriority=Speed
      settings: InputPortMap=u0
  Lookup_Mass : Interpolation_n-D  NumberOfTableDimensions=1  Table=PrelookupData.Tables.Mass  ExtrapMethod=Clip  DiagnosticForOutOfRangeInput=Warning  RequireIndexFractionAsBus=on  OutDataTypeStr=double  InternalRulePriority=Speed  TableDataTypeStr=Inherit: Inherit from 'Table data'
      settings: InputPortMap=u0
  Prelookup : PreLookup  BreakpointsData=PrelookupData.Breakpoints.Index  OutputSelection=Index and fraction as bus  IndexSearchMethod=Evenly spaced points
  TimeToIndex : Subsystem
  dIdt_Tensor(3x3) : Outport
  MOI_Tensor(3x3) : Outport  Port=2
  mass : Outport  Port=3
  COM_X : Outport  Port=4
  wires:
  Lookup_Mass/1 -> mass/1
  t/1 -> TimeToIndex/1(t)
  Lookup_COM_X/1 -> COM_X/1
  Direct Lookup Table (n-D)/1 -> Display/1, MOI_Tensor(3x3)/1
  Direct Lookup Table (n-D)1/1 -> dIdt_Tensor(3x3)/1
  Prelookup/1 -> Lookup_Mass/1, Lookup_COM_X/1
  TimeToIndex/1(Index) -> Direct Lookup Table (n-D)/1, Direct Lookup Table (n-D)1/1, Prelookup/1

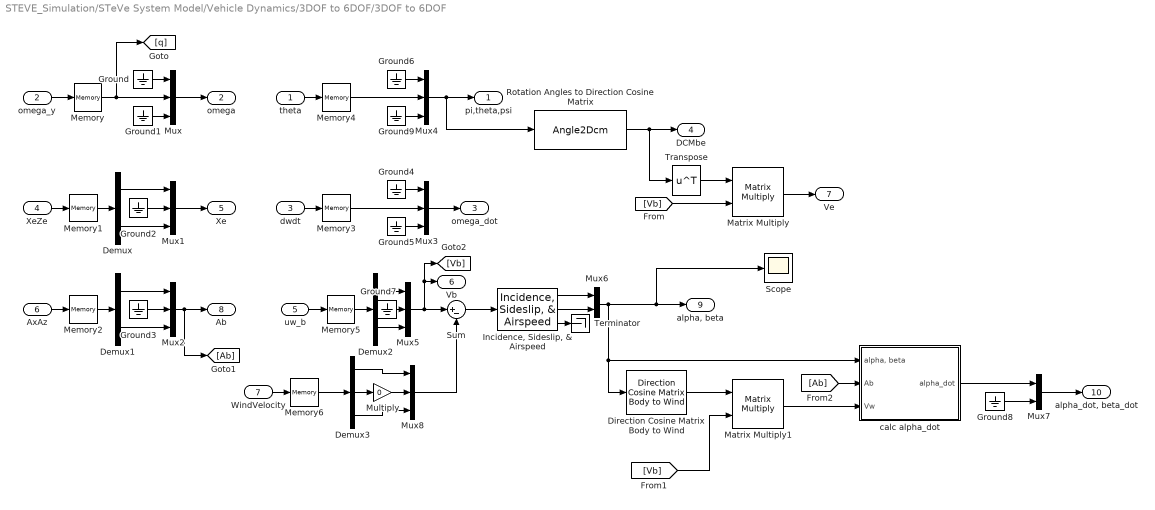
== system STEVE_Simulation/STeVe System Model/Vehicle Dynamics/3DOF to 6DOF/3DOF to 6DOF ==
  theta : Inport
  omega_y : Inport  Port=2
  dwdt : Inport  Port=3
  XeZe : Inport  Port=4
  uw_b : Inport  Port=5
  AxAz : Inport  Port=6
  WindVelocity : Inport  Port=7
  Demux : Demux  Outputs=2
  Demux1 : Demux  Outputs=2
  Demux2 : Demux  Outputs=2
  Demux3 : Demux  Outputs=3
  Direction Cosine Matrix Body to Wind : aerolibtransform2/Direction Cosine Matrix Body to Wind
  Ground{,1..9} (10 alike) : Ground
  "Incidence, Sideslip, & Airspeed" : aerolibasang/Incidence, Sideslip, & Airspeed
  Matrix Multiply : Product  Multiplication=Matrix(*)
  Matrix Multiply1 : Product  Multiplication=Matrix(*)
  Memory{,1..3,5..6} (6 alike) : Memory
  Memory4 : Memory  InitialCondition=Initial.Conditions.theta0
  Multiply : Gain  Gain=0
  Mux{,1..5,8} (7 alike) : Mux  Inputs=3
  Mux6 : Mux  Inputs=2
  Mux7 : Mux  Inputs=2
  Rotation Angles to Direction Cosine Matrix : Angle2Dcm
      settings: AttributesFormatString=Rotation Order: %<rotationOrder>
      mask Display:
      | port_label('input',1,'[R_1,R_2,R_3]','texmode','on')
      | port_label('output',1,'DCM_{be}','texmode','on')
  Scope : Scope
  Sum : Sum  Inputs=|+-
  Terminator : Terminator
  Transpose : Math  Operator=transpose
  calc alpha_dot : Subsystem
  pi,theta,psi : Outport
  omega : Outport  Port=2
  omega_dot : Outport  Port=3
  DCMbe : Outport  Port=4
  Xe : Outport  Port=5
  Vb : Outport  Port=6
  Ve : Outport  Port=7
  Ab : Outport  Port=8
  "alpha, beta" : Outport  Port=9
  "alpha_dot, beta_dot" : Outport  Port=10
  wires:
  omega_y/1 -> Memory/1
  Memory/1 -> [q], Mux/2
  Ground/1 -> Mux/1
  Ground1/1 -> Mux/3
  Demux/1 -> Mux1/1
  Ground2/1 -> Mux1/2
  Demux/2 -> Mux1/3
  Mux/1 -> omega/1
  XeZe/1 -> Memory1/1
  Memory1/1 -> Demux/1
  Mux1/1 -> Xe/1
  AxAz/1 -> Memory2/1
  Demux1/1 -> Mux2/1
  Demux1/2 -> Mux2/3
  Mux2/1 -> [Ab], Ab/1
  Memory2/1 -> Demux1/1
  Ground3/1 -> Mux2/2
  dwdt/1 -> Memory3/1
  Ground4/1 -> Mux3/1
  Ground5/1 -> Mux3/3
  Mux3/1 -> omega_dot/1
  Memory3/1 -> Mux3/2
  Ground9/1 -> Mux4/3
  Ground6/1 -> Mux4/1
  Mux4/1 -> Rotation Angles to Direction Cosine Matrix/1, pi,theta,psi/1
  theta/1 -> Memory4/1
  Memory4/1 -> Mux4/2
  Rotation Angles to Direction Cosine Matrix/1 -> Transpose/1, DCMbe/1
  Transpose/1 -> Matrix Multiply/1
  [Vb] -> Matrix Multiply/2
  Matrix Multiply/1 -> Ve/1
  uw_b/1 -> Memory5/1
  Demux2/2 -> Mux5/3
  Mux5/1 -> Sum/1, Vb/1, [Vb]
  Demux2/1 -> Mux5/1
  Ground7/1 -> Mux5/2
  Memory5/1 -> Demux2/1
  "Incidence, Sideslip, & Airspeed"/3 -> Terminator/1
  "Incidence, Sideslip, & Airspeed"/1 -> Mux6/1
  "Incidence, Sideslip, & Airspeed"/2 -> Mux6/2
  Mux6/1 -> calc alpha_dot/1("alpha, beta"), Direction Cosine Matrix Body to Wind/1, Scope/1, "alpha, beta"/1
  [Vb] -> Matrix Multiply1/2
  Direction Cosine Matrix Body to Wind/1 -> Matrix Multiply1/1
  Matrix Multiply1/1 -> calc alpha_dot/3(Vw)
  [Ab] -> calc alpha_dot/2(Ab)
  calc alpha_dot/1(alpha_dot) -> Mux7/1
  Ground8/1 -> Mux7/2
  Mux7/1 -> "alpha_dot, beta_dot"/1
  Sum/1 -> "Incidence, Sideslip, & Airspeed"/1
  WindVelocity/1 -> Memory6/1
  Memory6/1 -> Demux3/1
  Demux3/1 -> Mux8/1
  Multiply/1 -> Mux8/2
  Demux3/2 -> Multiply/1
  Demux3/3 -> Mux8/3
  Mux8/1 -> Sum/2

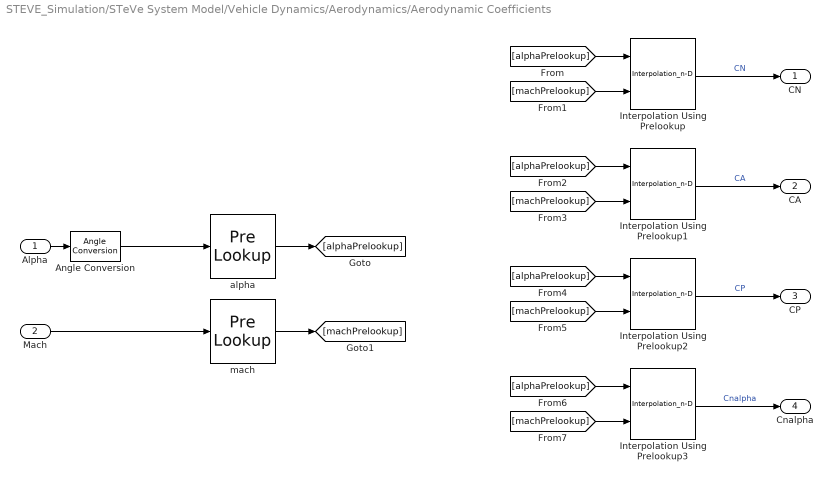
== system STEVE_Simulation/STeVe System Model/Vehicle Dynamics/Aerodynamics/Aerodynamic Coefficients ==
  Alpha : Inport
  Mach : Inport  Port=2
  Angle Conversion : aerolibconvert2/Angle Conversion  IU=rad  OU=deg
  Interpolation Using Prelookup : Interpolation_n-D  Table=AeroData.Tables.CN  RequireIndexFractionAsBus=on  InternalRulePriority=Speed
      settings: InputPortMap=u0,u1
  Interpolation Using Prelookup1 : Interpolation_n-D  Table=AeroData.Tables.CAPower_On  RequireIndexFractionAsBus=on  InternalRulePriority=Speed
      settings: InputPortMap=u0,u1
  Interpolation Using Prelookup2 : Interpolation_n-D  Table=AeroData.Tables.CP  RequireIndexFractionAsBus=on  InternalRulePriority=Speed
      settings: InputPortMap=u0,u1
  Interpolation Using Prelookup3 : Interpolation_n-D  Table=AeroData.Tables.Cnalpha  RequireIndexFractionAsBus=on  InternalRulePriority=Speed
      settings: InputPortMap=u0,u1
  alpha : PreLookup  BreakpointsData=AeroData.Breakpoints.Alpha  OutputSelection=Index and fraction as bus  IndexSearchMethod=Evenly spaced points  UseLastBreakpoint=on
  mach : PreLookup  BreakpointsData=AeroData.Breakpoints.Mach  OutputSelection=Index and fraction as bus  IndexSearchMethod=Evenly spaced points  ExtrapMethod=Linear
  CN : Outport
  CA : Outport  Port=2
  CP : Outport  Port=3
  Cnalpha : Outport  Port=4
  wires:
  Interpolation Using Prelookup/1 -> CN/1  "CN"
  alpha/1 -> [alphaPrelookup]
  mach/1 -> [machPrelookup]
  [alphaPrelookup] -> Interpolation Using Prelookup/1
  [machPrelookup] -> Interpolation Using Prelookup/2
  Interpolation Using Prelookup1/1 -> CA/1  "CA"
  [machPrelookup] -> Interpolation Using Prelookup1/2
  [alphaPrelookup] -> Interpolation Using Prelookup1/1
  Interpolation Using Prelookup2/1 -> CP/1  "CP"
  [machPrelookup] -> Interpolation Using Prelookup2/2
  [alphaPrelookup] -> Interpolation Using Prelookup2/1
  Interpolation Using Prelookup3/1 -> Cnalpha/1  "Cnalpha"
  [machPrelookup] -> Interpolation Using Prelookup3/2
  [alphaPrelookup] -> Interpolation Using Prelookup3/1
  Alpha/1 -> Angle Conversion/1
  Angle Conversion/1 -> alpha/1
  Mach/1 -> mach/1

== system STEVE_Simulation/STeVe System Model/Vehicle Dynamics/Aerodynamics/DerivedConditions ==
  Speed of sound : Inport
  Air Density : Inport  Port=2
  WindVelocity : Inport  Port=3
  WindAngularRates : Inport  Port=4
  Vb : Inport  Port=5
  Dot Product : DotProduct  OutDataTypeStr=Inherit: Inherit via internal rule
  Dynamic Pressure : aerolibasang/Dynamic Pressure
  Mach Number : aerolibasang/Mach Number
  Sqrt : Sqrt
  Sum : Sum  Inputs=|++
  Mach : Outport
  qbar : Outport  Port=2
  pqrWind : Outport  Port=3
  Airspeed : Outport  Port=4
  wires:
  WindVelocity/1 -> Sum/2
  Vb/1 -> Sum/1
  Speed of sound/1 -> Mach Number/2
  Sum/1 -> Dynamic Pressure/1, Mach Number/1, Dot Product/2, Dot Product/1
  Mach Number/1 -> Mach/1  "Mach"
  Air Density/1 -> Dynamic Pressure/2
  Dynamic Pressure/1 -> qbar/1  "qbar"
  WindAngularRates/1 -> pqrWind/1
  Dot Product/1 -> Sqrt/1
  Sqrt/1 -> Airspeed/1

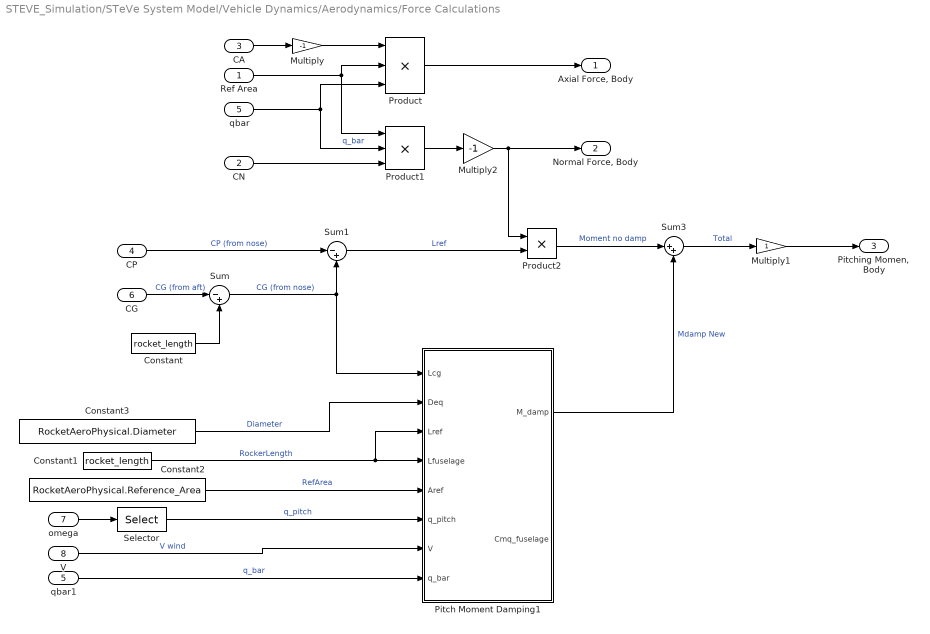
== system STEVE_Simulation/STeVe System Model/Vehicle Dynamics/Aerodynamics/Force Calculations ==
  Ref Area : Inport
  CN : Inport  Port=2
  CA : Inport  Port=3
  CP : Inport  Port=4
  qbar : Inport  Port=5
  CG : Inport  Port=6
  omega : Inport  Port=7
  V : Inport  Port=8
  Constant : Constant  Value=rocket_length
  Constant1 : Constant  Value=rocket_length
  Constant2 : Constant  Value=RocketAeroPhysical.Reference_Area
  Constant3 : Constant  Value=RocketAeroPhysical.Diameter  VectorParams1D=off
  Multiply : Gain  Gain=-1
  Multiply1 : Gain
  Multiply2 : Gain  Gain=-1
  Pitch Moment Damping1 : MATLAB Function  TreatAsAtomicUnit=on
  Product : Product  Inputs=***
  Product1 : Product  Inputs=***
  Product2 : Product
  Selector : Selector  InputPortWidth=3  IndexOptions=Index vector (dialog)  Indices=2  OutputSizes=1
  Sum : Sum  Inputs=|-+
  Sum1 : Sum  Inputs=|-+
  Sum3 : Sum  Inputs=|++
  qbar1 : InportShadow  Port=5
  "Axial Force, Body" : Outport
  "Normal Force, Body" : Outport  Port=2
  "Pitching Momen, Body" : Outport  Port=3
  wires:
  Product/1 -> "Axial Force, Body"/1
  CA/1 -> Multiply/1
  qbar/1 -> Product/3, Product1/2  "q_bar"
  Ref Area/1 -> Product/2, Product1/1
  Multiply/1 -> Product/1
  Product1/1 -> Multiply2/1
  CN/1 -> Product1/3
  CP/1 -> Sum1/1  "CP (from nose)"
  Sum1/1 -> Product2/2  "Lref"
  Product2/1 -> Sum3/1  "Moment no damp"
  Sum3/1 -> Multiply1/1  "Total"
  Sum/1 -> Pitch Moment Damping1/1(Lcg), Sum1/2  "CG (from nose)"
  Constant/1 -> Sum/2
  Multiply1/1 -> "Pitching Momen, Body"/1
  Multiply2/1 -> Product2/1, "Normal Force, Body"/1
  V/1 -> Pitch Moment Damping1/7(V)  "V wind"
  Constant2/1 -> Pitch Moment Damping1/5(Aref)  "RefArea"
  Constant1/1 -> Pitch Moment Damping1/3(Lref), Pitch Moment Damping1/4(Lfuselage)  "RockerLength"
  Constant3/1 -> Pitch Moment Damping1/2(Deq)  "Diameter"
  omega/1 -> Selector/1
  Selector/1 -> Pitch Moment Damping1/6(q_pitch)  "q_pitch"
  qbar1/1 -> Pitch Moment Damping1/8(q_bar)  "q_bar"
  CG/1 -> Sum/1  "CG (from aft)"
  Pitch Moment Damping1/1(M_damp) -> Sum3/2  "Mdamp New"

== system STEVE_Simulation/STeVe System Model/Vehicle Dynamics/Propulsion F,M/Subsystem ==
  Thrust : Inport
  Nozzle Angle : Inport  Port=2
  CG : Inport  Port=3
  Cos : Trigonometry  Operator=cos
  Product : Product
  Product1 : Product  OutDataTypeStr=double
  Product2 : Product
  Sin : Trigonometry
  Ft_x_b : Outport
  Ft_z_b : Outport  Port=2
  M_y_b : Outport  Port=3
  wires:
  Nozzle Angle/1 -> Sin/1, Cos/1
  Thrust/1 -> Product1/1, Product/1
  Product/1 -> Ft_x_b/1
  Cos/1 -> Product/2
  Product1/1 -> Product2/1, Ft_z_b/1
  Sin/1 -> Product1/2
  Product2/1 -> M_y_b/1
  CG/1 -> Product2/2

== system STEVE_Simulation/STeVe System Model/Vehicle Dynamics/Time Varying Parameters/TimeToIndex ==
  t : Inport
  Add Constant : Bias  Bias=1  SaturateOnIntegerOverflow=off
  Constant : Constant  Value=timeStep
  Product : Product  Inputs=*/
  Index : Outport
  wires:
  t/1 -> Product/1
  Constant/1 -> Product/2
  Product/1 -> Add Constant/1
  Add Constant/1 -> Index/1

== system STEVE_Simulation/STeVe System Model/Vehicle Dynamics/3DOF to 6DOF/3DOF to 6DOF/calc alpha_dot ==
  "alpha, beta" : Inport
  Ab : Inport  Port=2
  Vw : Inport  Port=3
  "Add epsilon to avoid division by 0 " : Bias  Bias=1*10^-8  SaturateOnIntegerOverflow=off
  Direction Cosine Matrix Body to Wind : aerolibtransform2/Direction Cosine Matrix Body to Wind
  Matrix Multiply : Product  Multiplication=Matrix(*)
  Product : Product  Inputs=*/
  Selector : Selector  IndexMode=Zero-based  InputPortWidth=3  IndexOptions=Index vector (dialog)  Indices=2  OutputSizes=1
  Selector1 : Selector  IndexMode=Zero-based  InputPortWidth=3  IndexOptions=Index vector (dialog)  Indices=0  OutputSizes=1
  alpha_dot : Outport
  wires:
  "alpha, beta"/1 -> Direction Cosine Matrix Body to Wind/1
  Direction Cosine Matrix Body to Wind/1 -> Matrix Multiply/1
  Ab/1 -> Matrix Multiply/2
  Matrix Multiply/1 -> Selector/1
  Vw/1 -> Selector1/1
  Selector/1 -> Product/1
  Selector1/1 -> "Add epsilon to avoid division by 0 "/1
  Product/1 -> alpha_dot/1
  "Add epsilon to avoid division by 0 "/1 -> Product/2

== matlab function STEVE_Simulation/STeVe System Model/Vehicle Dynamics/RocketEngineActuators/MATLAB Function1 ==
  data: desired_nozzle_angle_rad input; delta_S_command output
function delta_S_command = inverse_kinematics_nozzle(desired_nozzle_angle_rad)
% Calculates the required linear actuator stroke (delta_S) for a desired
% nozzle deflection angle (desired_nozzle_angle_rad).
% desired_nozzle_angle_rad is the CHANGE in the angle between linkage arms
% from their initial configuration (when delta_S = 0).
%
% Input:
%   desired_nozzle_angle_rad: The desired change in nozzle angle, in RADIANS.
%
% Output:
%   delta_S_command: The required change in actuator length (stroke), in meters.

%#codegen % Required for Simulink code generation

% Linkage parameters (constants)
l = 0.173086;   % m (First arm length)
r = 0.187926;   % m (Second arm length)
S0 = 0.221779;  % m (Initial actuator length when desired_nozzle_angle_rad is 0)

% --- Calculate the initial internal angle based on S0, l, and r ---
% This is the angle between arms l and r when desired_nozzle_angle_rad is 0 (and delta_S is 0).
% cos(initial_internal_angle) = (l^2 + r^2 - S0^2) / (2 * l * r)
cos_arg_initial = (l^2 + r^2 - S0^2) / (2 * l * r);

% Clamp for safety, though with consistent S0, l, r, it should be valid
if cos_arg_initial > 1.0
    cos_arg_initial = 1.0;
elseif cos_arg_initial < -1.0
    cos_arg_initial = -1.0;
end
initial_internal_angle_rad = acos(cos_arg_initial);
% --------------------------------------------------------------------

% Calculate the target total internal angle for the linkage
% This is the initial angle PLUS the desired change.
target_total_internal_angle_rad = initial_internal_angle_rad + desired_nozzle_angle_rad;

% Calculate S_total_squared = (S0 + delta_S)^2 using the law of cosines
% for the target_total_internal_angle_rad
S_total_squared = l^2 + r^2 - 2*l*r*cos(target_total_internal_angle_rad);

% --- Handle Physical Impossibility (Saturation) ---
% S_total_squared should theoretically be between (l-r)^2 and (l+r)^2.
% (l-r)^2 corresponds to the arms being collinear and extended in opposite directions (shortest S).
% (l+r)^2 corresponds to the arms being collinear and extended in the same direction (longest S).
S_min_possible_squared = (l-r)^2;
S_max_possible_squared = (l+r)^2;

if S_total_squared < S_min_possible_squared
    % This can happen if target_total_internal_angle_rad is too close to 0 or pi (collinear)
    % and the desired S is shorter than physically possible.
    % Or due to floating point errors if very close to the limit.
    coder.varsize('warning_text_min', [1, 200]);
    warning_text_min = sprintf('Warning: Desired angle (%.2f rad from initial) leads to S_total_squared (%.4e) < S_min_possible_squared (%.4e). Clamping.', desired_nozzle_angle_rad, S_total_squared, S_min_possible_squared);
    warning(warning_text_min);
    S_total_squared = S_min_possible_squared;
elseif S_total_squared > S_max_possible_squared
    % This implies the angle is such that it requires S > l+r, which is impossible.
    coder.varsize('warning_text_max', [1, 200]);
    warning_text_max = sprintf('Warning: Desired angle (%.2f rad from initial) leads to S_total_squared (%.4e) > S_max_possible_squared (%.4e). Clamping.', desired_nozzle_angle_rad, S_total_squared, S_max_possible_squared);
    warning(warning_text_max);
    S_total_squared = S_max_possible_squared;
end
% An additional check if S_total_squared somehow still ended up negative, though the above should prevent it.
if S_total_squared < 0
    S_total_squared = 0; % Fallback, should ideally be S_min_possible_squared
end
% --- End Handle Physical Impossibility ---

% Calculate the total desired actuator length S_total = S0 + delta_S
S_total_desired = sqrt(S_total_squared);

% Calculate the required actuator stroke delta_S
delta_S_command = S_total_desired - S0;

end

== matlab function STEVE_Simulation/Environment/g(h) ==
  data: h input; g output
function g = fcn(h)
G = 6.67430*10^(-11);
M = 5.9722*10^(24);
R_e = 6.371*10^(6);

g = (G * M)/(R_e + h)^2;
